simulink model "laserscan2templateMatchPolygon"  (R2016a)
settings: Solver=FixedStepAuto  StartTime=0.0  StopTime=inf  FixedStep=1.0  RelTol=1e-3
model workspace (MAT data in the model file):
  SL_ROS_VariableLengthArrays_MaxSizes.CommonInfo.ArrayTruncateAction = 'EmitWarning'
  SL_ROS_VariableLengthArrays_MaxSizes.MsgTypeMap = containers.Map
  SL_ROS_VariableLengthArrays_MaxSizes.MsgTypeMap.serialization.keys = {'sensor_msgs/LaserScan'}
  SL_ROS_VariableLengthArrays_MaxSizes.MsgTypeMap.serialization.values{1}(1).PropertyName = 'Ranges'
  SL_ROS_VariableLengthArrays_MaxSizes.MsgTypeMap.serialization.values{1}(1).DataType = 'single'
  SL_ROS_VariableLengthArrays_MaxSizes.MsgTypeMap.serialization.values{1}(1).MaxLength = 180
  SL_ROS_VariableLengthArrays_MaxSizes.MsgTypeMap.serialization.values{1}(2).PropertyName = 'Intensities'
  SL_ROS_VariableLengthArrays_MaxSizes.MsgTypeMap.serialization.values{1}(2).DataType = 'single'
  SL_ROS_VariableLengthArrays_MaxSizes.MsgTypeMap.serialization.values{1}(2).MaxLength = 180
  SL_ROS_VariableLengthArrays_MaxSizes.MsgTypeMap.serialization.uniformity = 0
  SL_ROS_VariableLengthArrays_MaxSizes.MsgTypeMap.serialization.keyType = 'char'
  SL_ROS_VariableLengthArrays_MaxSizes.MsgTypeMap.serialization.valueType = 'any'
undefined symbols (not defined in the file): Header, Rec, SDTV
libraries: robotlib x4, visionconversions x3, visionsinks x2, visiontextngfix x1, visionsources x1, visionanalysis x1
settings Model: Creator=sprinkle  LastModifiedBy=sprinkle
settings OptimizationCC: OptimizeModelRefInitCode=on  LifeSpan=Inf  MaxStackSize=64
settings HardwareCC: ProdBitPerPointer=32  ProdLargestAtomicFloat=None  ProdIntDivRoundTo=Undefined  ProdEndianess=Unspecified  ProdWordSize=32  ProdHWDeviceType=Generic->Unspecified (assume 32-bit Generic)
settings RTWCC: SystemTargetFile=ert.tlc  HardwareBoard=Robot Operating System (ROS)  TemplateMakefile=ert_default_tmf  GenerateReport=on  Toolchain=Catkin  IncludeHyperlinkInReport=on  LaunchReport=on  TargetLang=C++  GenerateTraceInfo=on  GenerateTraceReport=on  GenerateTraceReportSl=on  GenerateTraceReportSf=on  GenerateTraceReportEml=on
settings CodeAppCC: ForceParamTrailComments=on  IgnoreCustomStorageClasses=off  OperatorAnnotations=on  SimulinkDataObjDesc=on  SFDataObjDesc=on  MATLABFcnDesc=on  InsertBlockDesc=on  MATLABSourceComments=on
settings ERTTargetCC: SupportVariableSizeSignals=on

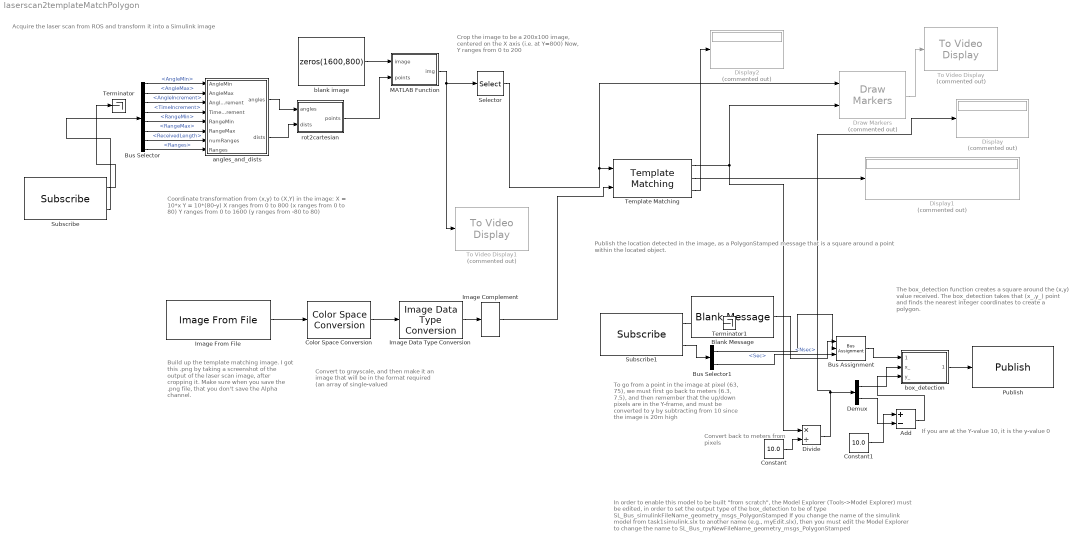
== system laserscan2templateMatchPolygon ==
  note: Crop the image to be a 200x100 image, centered on the X axis (i.e. at Y=800)
      |
      | Now, Y ranges from 0 to 200
  note: Coordinate transformation from (x,y) to (X,Y) in the image:
      |   X = 10*x
      |   Y = 10*(80-y)
      | X ranges from 0 to 800 (x ranges from 0 to 80)
      | Y ranges from 0 to 1600 (y ranges from -80 to 80)
  note: To go from a point in the image at pixel (63, 75), we must first go back to meters (6.3, 7.5), and then remember that the up/down pixels are in the Y-frame, and must be converted to y by subtracting from 10 since the image is 20m high
  note: Convert back
      | to meters from pixels
  note: Convert to grayscale, and then make it an image that will be in the format required (an array of single-valued
  note: Acquire the laser scan from ROS and transform it into a Simulink image
  note: In order to enable this model to be built "from scratch", the Model Explorer (Tools->Model Explorer) must be
      | edited, in order to set the output type of the box_detection to be of type
      | SL_Bus_simulinkFileName_geometry_msgs_PolygonStamped
      | If you change the name of the simulink model from task1simulink.slx to another name (e.g., myEdit.slx),
      | then you must edit the Model Explorer to change the name to
      | SL_Bus_myNewFileName_geometry_msgs_PolygonStamped
  note: The box_detection function creates a square around the (x,y) value received. The box_detection takes that (x_,y_) point and finds the nearest integer coordinates to create a polygon.
  note: Publish the location detected in the image, as a PolygonStamped message that is a square around a point within the located object.
  note: Build up the template matching image. I got this .png by taking a screenshot of the output of the laser scan image, after cropping it. Make sure when you save the .png file, that you don't save the Alpha channel.
  note: If you are at the Y-value 10, it is the y-value 0
  Add : Sum  Inputs=+-
  Blank Message : robotlib/Blank Message  SourceLibraryInfo=This block requires Robotics System Toolbox  messageType=geometry_msgs/PolygonStamped  SampleTime=inf
  Bus Assignment : BusAssignment  AssignedSignals=Header.Stamp.Sec,Header.Stamp.Nsec
  Bus Selector : BusSelector  OutputSignals=AngleMin,AngleMax,AngleIncrement,TimeIncrement,RangeMin,RangeMax,Ranges_SL_Info.ReceivedLength,Ranges
  Bus Selector1 : BusSelector  OutputSignals=Clock_.Sec,Clock_.Nsec
  Color Space Conversion : visionconversions/Color Space  Conversion  conversion=Obsolete  conversionActive=R'G'B' to intensity  wp_str=D65  rec=Rec. 601 (SDTV)  sys=1125/60/2:1  imagePorts=One multidimensional signal
  Constant : Constant  Value=10.0
  Constant1 : Constant  Value=10.0
  Demux : Demux  Outputs=2
  Display : Display  Commented=on
  Display1 : Display  Commented=on
  Display2 : Display  Commented=on
  Divide : Product  Inputs=*/
  Draw Markers : visiontextngfix/Draw Markers  Commented=on  shape=Circle  size=30  fill=on  fillClrSource=Specify via dialog  display=White  intensity=200  color=[200 255 100]  opacity=0.6  viewport=Entire image  antialiasing=off  inType=Obsolete  imagePorts=One multidimensional signal  prodOutputMode=Binary point scaling  prodOutputWordLength=32  prodOutputFracLength=14  memoryMode=Specify word length  memoryWordLength=16  memoryFracLength=14  roundingMode=Floor  overflowMode=off
  Image Complement : visionconversions/Image Complement
  Image Data Type Conversion : visionconversions/Image Data Type Conversion  outDT=single  isSigned=on  wordLen=16  numFracBits=0
  Image From File : visionsources/Image From File  Tag=vipblks_nd  FileName=/home/sprinkle/Pictures/barrel.png  imagePorts=One multidimensional signal  Ts=inf  ImageDataType=Inherit from input image  Signed=on  WordLength=16  sdImageDataType=uint(8)  FractionLengthMode=User-defined  FractionLength=15  OutPortLabels=R|G|B
  MATLAB Function : MATLAB Function  TreatAsAtomicUnit=on
  Publish : robotlib/Publish  SourceLibraryInfo=This block requires Robotics System Toolbox  topicSource=Specify your own  topic=/detections  messageType=geometry_msgs/PolygonStamped  messageQueueLength=1
  Selector : Selector  NumberOfDimensions=2  InputPortWidth=3  IndexOptions=Starting index (dialog),Starting index (dialog)  Indices=700,1  OutputSizes=200,100
  Subscribe : robotlib/Subscribe  SourceLibraryInfo=This block requires Robotics System Toolbox  topicSource=Select from ROS network  topic=/catvehicle/front_laser_points  messageType=sensor_msgs/LaserScan  sampleTime=-1  messageQueueLength=1
  Subscribe1 : robotlib/Subscribe  SourceLibraryInfo=This block requires Robotics System Toolbox  topicSource=Select from ROS network  topic=/clock  messageType=rosgraph_msgs/Clock  sampleTime=-1  messageQueueLength=1
  Template Matching : visionanalysis/Template Matching  metric=Sum of squared differences  output=Best match location  method=Exhaustive  nMetric=on  nSize=3  roi=off  roiValid=off  accumMode=Binary point scaling  accumWordLength=32  accumFracLength=0  prodOutputMode=Binary point scaling  prodOutputWordLength=32  prodOutputFracLength=0  roundingMode=Floor  overflowMode=off
  Terminator : Terminator
  Terminator1 : Terminator
  To Video Display : visionsinks/To Video Display  Commented=on  windowSizeMode=Normal  openAtMdlStart=on  fullScreen=off  videoWindowX=1310  videoWindowY=476  saveWindowSize=off  videoWindowWidth=378  videoWindowHeight=413  inputColorFormat=RGB  inputType=Obsolete  imagePorts=One multidimensional signal  OutputDevice=On-screen video monitor  dataOrg=Column-major  isWindowOpen=off
  To Video Display1 : visionsinks/To Video Display  Commented=on  windowSizeMode=Normal  openAtMdlStart=on  fullScreen=off  videoWindowX=500  videoWindowY=239  saveWindowSize=off  videoWindowWidth=479  videoWindowHeight=843  inputColorFormat=RGB  inputType=Obsolete  imagePorts=One multidimensional signal  OutputDevice=On-screen video monitor  dataOrg=Column-major  isWindowOpen=off
  angles_and_dists : MATLAB Function  TreatAsAtomicUnit=on
  blank image : Constant  Value=zeros(1600,800)
  box_detection : MATLAB Function  TreatAsAtomicUnit=on
  rot2cartesian : MATLAB Function  TreatAsAtomicUnit=on
  wires:
  Subscribe/1 -> Terminator/1
  Subscribe/2 -> Bus Selector/1
  Bus Selector/1 -> angles_and_dists/1(AngleMin)  "<AngleMin>"
  Bus Selector/2 -> angles_and_dists/2(AngleMax)  "<AngleMax>"
  Bus Selector/3 -> angles_and_dists/3(AngleIncrement)  "<AngleIncrement>"
  Bus Selector/4 -> angles_and_dists/4(TimeIncrement)  "<TimeIncrement>"
  Bus Selector/5 -> angles_and_dists/5(RangeMin)  "<RangeMin>"
  Bus Selector/6 -> angles_and_dists/6(RangeMax)  "<RangeMax>"
  Bus Selector/7 -> angles_and_dists/7(numRanges)  "<ReceivedLength>"
  Bus Selector/8 -> angles_and_dists/8(Ranges)  "<Ranges>"
  angles_and_dists/1(angles) -> rot2cartesian/1(angles)
  angles_and_dists/2(dists) -> rot2cartesian/2(dists)
  rot2cartesian/1(points) -> MATLAB Function/2(points)
  blank image/1 -> MATLAB Function/1(image)
  MATLAB Function/1(img) -> To Video Display1/1, Selector/1
  Template Matching/1 -> Divide/1, Draw Markers/2
  Image From File/1 -> Color Space Conversion/1
  Color Space Conversion/1 -> Image Data Type Conversion/1
  Draw Markers/1 -> To Video Display/1
  Template Matching/2 -> Display1/1
  Template Matching/3 -> Display2/1
  Image Data Type Conversion/1 -> Image Complement/1
  Image Complement/1 -> Template Matching/2
  Selector/1 -> Draw Markers/1, Template Matching/1
  Blank Message/1 -> Bus Assignment/1
  box_detection/1(outputMsg) -> Publish/1
  Bus Assignment/1 -> box_detection/1(blankMsg)
  Demux/1 -> box_detection/2(x_)
  Subscribe1/1 -> Terminator1/1
  Subscribe1/2 -> Bus Selector1/1
  Bus Selector1/1 -> Bus Assignment/2  "<Sec>"
  Bus Selector1/2 -> Bus Assignment/3  "<Nsec>"
  Divide/1 -> Display/1, Demux/1
  Constant/1 -> Divide/2
  Add/1 -> box_detection/3(y_)
  Constant1/1 -> Add/1
  Demux/2 -> Add/2

== matlab function laserscan2templateMatchPolygon/rot2cartesian ==
  data: angles input; dists input; points output size=[180 2]
function points = fcn(angles,dists)
%#codegen
xs = dists.*cos(angles);
ys = dists.*sin(angles);
points = [xs,ys];

== matlab function laserscan2templateMatchPolygon/angles_and_dists ==
  data: AngleMin input size=1 [-2*pi..2*pi]; angles output size=[180 1]; dists output size=[180 1]; AngleMax input [-2*pi..2*pi]; AngleIncrement input [0..2*pi]; TimeIncrement input; RangeMin input; RangeMax input; numRanges input [1..360]; Ranges input
function [angles,dists] = fcn(AngleMin, AngleMax, AngleIncrement, ...
                TimeIncrement, RangeMin, RangeMax, numRanges, Ranges )
%#codegen
% this function transforms the laser scan into cartesian coordinates, so
% that you can use other tools to group them together, make an image, etc.
if numRanges > 0 
angleMin = double(AngleMin);
angleMax = double(AngleMax);
angleIncrement = double(AngleIncrement);
% assert(angleMax > angleMin);
% assert((angleMax-angleMin)/angleIncrement > 1);

angleMin = -pi/2;
angleMax = pi/2;
angleIncrement = pi/179;
timeIncrement = TimeIncrement;
rangeMin = RangeMin;
rangeMax = RangeMax;
ranges = Ranges;
ranges(ranges>RangeMax) = NaN;
ranges(ranges<RangeMin) = NaN;
%rangesLength = scan.Ranges_SL_Info.ReceivedLength;
%intensities = scan.Intensities;
%coder.varsize('angles',[180 1]);
assert(numRanges < 360);
angles=double(zeros(numRanges,1));
for ii=1:numRanges
    angles(ii) = double(angleMin) + double(ii-1)*(angleIncrement);
end
% angles = [angleMin:angleIncrement:angleMax]';
dists = ranges;
assert(length(dists) == numRanges);
assert(length(dists) == length(angles));
else
    angles=double(0);
    dists=single(0);
end

== matlab function laserscan2templateMatchPolygon/MATLAB Function ==
  data: image input; img output; points input size=[180 2]
function img = fcn(image,points)
%#codegen
img = single(image);
% we assume we will be getting 180x2 points
len=180;
% the point (0,-20) would, normally, be in the bottom half of the image
% note: (with +x forward, and +y to the left of the car).
% But, the bottom half of the image should be +20 more pixels. So, we will
% instead /subtract/ from 80, all the points. That way, point
pts = points;
% add 80 to all the y points
pts(:,2) = 80 - pts(:,2);
% since we are building an 800x1600 image of the 80m (x) by 160m (y), we
% will multiply the data by 10 and take the floor in order to show
% occupancy near that point
pts = single(10*pts);
% iterate over these points, and set up a primitive grid map
for ii=1:len
    ii_x = pts(ii,1); % the x point is in the first column
    ii_y = pts(ii,2); % the y point is in the second comlumn
    if(ii_x > 800)
        disp('ru roh');
    end
    index_x = min(max(10,floor(ii_x)),800-10);
    index_y = min(max(10,floor(ii_y)),1600-10);
    % make a square here, of size 10x10 pixels
    % we must swap the (x,y) to (y,x) for MATLAB images
    img(index_y-5:index_y+5,index_x-5:index_x+5) = ...
        img(index_y-5:index_y+5,index_x-5:index_x+5) | 255;
end

== matlab function laserscan2templateMatchPolygon/box_detection ==
  data: blankMsg input; x_ input; outputMsg output Bus: SL_Bus_laserscan2templateMatchPo_PolygonStamped_el3kzr; y_ input
    function outputMsg = fcn(blankMsg,x_,y_)
    %#codegen
    % the sequence of the message must increment each time we publish, so we
    % need it to be persistent across instantiations
    persistent seq;

    % if this is the first time our model is run, then 'seq' will not exist.
    % Then 'isempty(seq)' will be true, which allows us to intialize it to 0
    if isempty(seq)
        seq=uint32(0);
    end

    % increment the sequence number
    seq = seq+1;
    % set our output to be a copy of the input (blankMsg)
    outputMsg = blankMsg;
    % these points in (x,y,z) are either taken from the inputs, or hardcoded
    x = single(x_);
    y = single(y_);
    z = single(0);
    % by definition in this block, we are making a square.
    % IF YOU USE THIS model as inspiration for an output detection that is a
    % pentagon, then you would set the length to be 5, for example.
    outputMsg.Polygon.Points_SL_Info.CurrentLength = uint32(4);
    % set the frame to be relative to our base of 0. If you want to use data
    % coming from another detection, then you can set the /detections to be in
    % the frame of that specific sensor
    str = 'catvehicle/front_laser_link';
    % initialize the header and set its values
    strLength = length(str);
    outputMsg.Header.Seq = seq;
    outputMsg.Header.FrameId(1:strLength) = str;
    outputMsg.Header.FrameId_SL_Info.CurrentLength = uint32(strLength);

    % populate point 1
    outputMsg.Polygon.Points(1).X = floor(x);
    outputMsg.Polygon.Points(1).Y = floor(y);
    outputMsg.Polygon.Points(1).Z = z;

    % populate point 2
    outputMsg.Polygon.Points(2).X = floor(x);
    outputMsg.Polygon.Points(2).Y = ceil(y);
    outputMsg.Polygon.Points(2).Z = z;

    % populate point 3
    outputMsg.Polygon.Points(3).X = ceil(x);
    outputMsg.Polygon.Points(3).Y = ceil(y);
    outputMsg.Polygon.Points(3).Z = z;

    % populate point 4
    outputMsg.Polygon.Points(4).X = ceil(x);
    outputMsg.Polygon.Points(4).Y = floor(y);
    outputMsg.Polygon.Points(4).Z = z;

    % note that the polygon type "closes" between the last and first points
